simulink model "ego"  (R2024b)
settings: Solver=FixedStepAuto  StartTime=0.0  StopTime=5  RelTol=1e-3
settings Model: Creator=DELL  LastModifiedBy=DELL

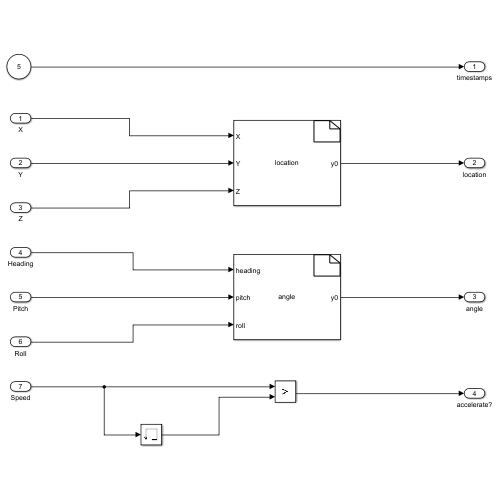
[thumbnail: Simulink's stored preview of the top-level diagram]
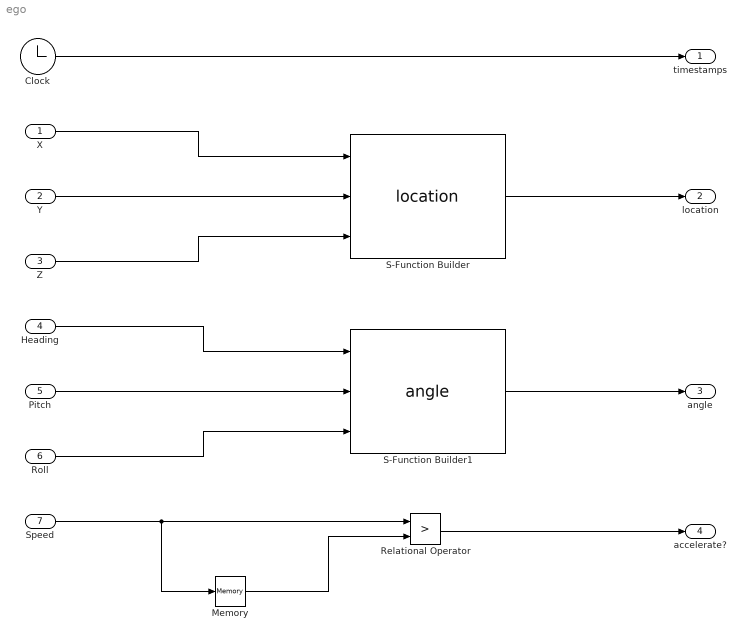
== system ego ==
  X : Inport  Tag=X
  Y : Inport  Tag=Y  Port=2
  Z : Inport  Tag=Z  Port=3
  Heading : Inport  Tag=Heading  Port=4
  Pitch : Inport  Tag=Pitch  Port=5
  Roll : Inport  Tag=Roll  Port=6
  Speed : Inport  Tag=Speed  Port=7
  Clock : Clock
  Memory : Memory  LinearizeAsDelay=on
  Relational Operator : RelationalOperator  Operator=>  OutDataTypeStr=boolean  RndMeth=Simplest  InputSameDT=off
  S-Function Builder : S-Function  FunctionName=location  SFunctionModules=location_wrapper.cpp  SFunctionDeploymentMode=off  EnableBusSupport=off  mask(S-Function Builder){}
      mask help: Simulink:masks:SFunctionBuilder_MD
      mask init:
      | val = [[.9  0.75 0.75 1 1 .9 .9 1]',[1 1 0.75 0.75 .9 .9 1 .9]'];try , sys = get_param(gcb,'SfunBuilderFcnName');if isempty(sys), sys = get_param(gcb,'FunctionName'); end,catch, sys = get_param(gcb,'FunctionName'); end
      settings: CopyFcn=set_param(gcbh,'LinkStatus','none')  OpenFcn=sfunctionwizard(gcbh)
      mask Display:
      | plot(val(:,1),val(:,2))
      | disp(sys)
      | port_label('input',1,sprintf('%s', 'X'),'interpreter','tex')
      | port_label('input',2,sprintf('%s', 'Y'),'interpreter','tex')
      | port_label('input',3,sprintf('%s', 'Z'),'interpreter','tex')
      | port_label('output',1,sprintf('%s', 'y0'),'interpreter','tex')
  S-Function Builder1 : S-Function  FunctionName=angle  SFunctionModules=angle_wrapper.cpp  SFunctionDeploymentMode=off  EnableBusSupport=off  mask(S-Function Builder){}
      mask help: Simulink:masks:SFunctionBuilder_MD
      mask init: same as ego/S-Function Builder
      settings: CopyFcn=set_param(gcbh,'LinkStatus','none')  OpenFcn=sfunctionwizard(gcbh)
      mask Display:
      | plot(val(:,1),val(:,2))
      | disp(sys)
      | port_label('input',1,sprintf('%s', 'heading'),'interpreter','tex')
      | port_label('input',2,sprintf('%s', 'pitch'),'interpreter','tex')
      | port_label('input',3,sprintf('%s', 'roll'),'interpreter','tex')
      | port_label('output',1,sprintf('%s', 'y0'),'interpreter','tex')
  timestamps : Outport
  location : Outport  Port=2
  angle : Outport  Port=3
  accelerate? : Outport  Port=4
  wires:
  X/1 -> S-Function Builder/1
  Y/1 -> S-Function Builder/2
  Z/1 -> S-Function Builder/3
  Heading/1 -> S-Function Builder1/1
  Pitch/1 -> S-Function Builder1/2
  Roll/1 -> S-Function Builder1/3
  Speed/1 -> Memory/1, Relational Operator/1
  Relational Operator/1 -> accelerate?/1
  Clock/1 -> timestamps/1
  S-Function Builder/1 -> location/1
  S-Function Builder1/1 -> angle/1
  Memory/1 -> Relational Operator/2
